simulink model "TwoTankSystem_continuous_controller"  (R2017a)
settings: Solver=ode4  StartTime=0.0  StopTime=SIM_TIME  FixedStep=STEP_SIZE  RelTol=1e-3  EnableMultiTasking=on
values from neighbouring files (symbols this model uses):
  At = 0.785    [TwoTankSystem.m]
  Av0 = 0.0122    [TwoTankSystem.m]
  Av1 = 1.2*0.0122    (= 0.01464)    [TwoTankSystem.m]
  B = B(:,1:2)    [TwoTankSystem.m]
  Bv = B(:,3:5)    [TwoTankSystem.m]
  C0 = 0.056    [TwoTankSystem.m]
  Dv = 2.66    [TwoTankSystem.m]
  K_CT = K_fs    [TwoTankSystem.m]
  ka = 0.004    [TwoTankSystem.m]
  kh = 2    [TwoTankSystem.m]
  kt = 0.1    [TwoTankSystem.m]
  r0 = [H_ref0 T_ref0]'    [TwoTankSystem.m]
  r1 = [0.5 -0.5]'    [TwoTankSystem.m]
  Tc = 1500    [TwoTankSystem.m]
  Tc0 = 30    [TwoTankSystem.m]
  Tc1 = 20    [TwoTankSystem.m]
  Tref1 = 100    [TwoTankSystem.m]
  Tref2 = 500    [TwoTankSystem.m]
  Tv = 2200    [TwoTankSystem.m]
  Tw = 300    [TwoTankSystem.m]
  Tw0 = 60    [TwoTankSystem.m]
  Tw1 = 75    [TwoTankSystem.m]
  u0 = u0(1:2,1)    [TwoTankSystem.m]
  v0 = u0(3:5,1)    [TwoTankSystem.m]
  x0 = xFinal'    [TwoTankSystem.m]
  x0_lin = zeros(size(A,1),1)    [TwoTankSystem.m]
  y0 = C*x0    [TwoTankSystem.m]
undefined symbols (not defined in the file or in its folder): A, C
settings Model: Creator=roga  LastModifiedBy=Roberto
settings DataIOCC: LimitDataPoints=on  SaveFinalState=on  SaveFormat=Array
settings OptimizationCC: LifeSpan=inf
settings DebuggingCC: UnderspecifiedInitializationDetection=Classic  MergeDetectMultiDrivingBlocksExec=none  SolverPrmCheckMsg=warning  StateNameClashWarn=warning  SFUnexpectedBacktrackingDiag=warning  SFNoUnconditionalDefaultTransitionDiag=warning  SFExecutionAtInitializationDiag=none
settings HardwareCC: ProdBitPerPointer=32  ProdBitPerSizeT=32  ProdBitPerPtrDiffT=32  ProdLargestAtomicFloat=None  ProdIntDivRoundTo=Undefined  ProdEndianess=Unspecified  ProdWordSize=32  ProdHWDeviceType=32-bit Generic
settings ModelReferenceCC: PropagateSignalLabelsOutOfModel=off
settings GRTTargetCC: TargetLangStandard=C89/C90 (ANSI)  GeneratePreprocessorConditionals=Disable all
settings ConfigComp: CovMetricSettings=dw  CovHtmlReporting=on  CovSaveCumulativeToWorkspaceVar=on  CovSaveSingleToWorkspaceVar=on  CovExternalEMLEnable=off  CovSFcnEnable=off

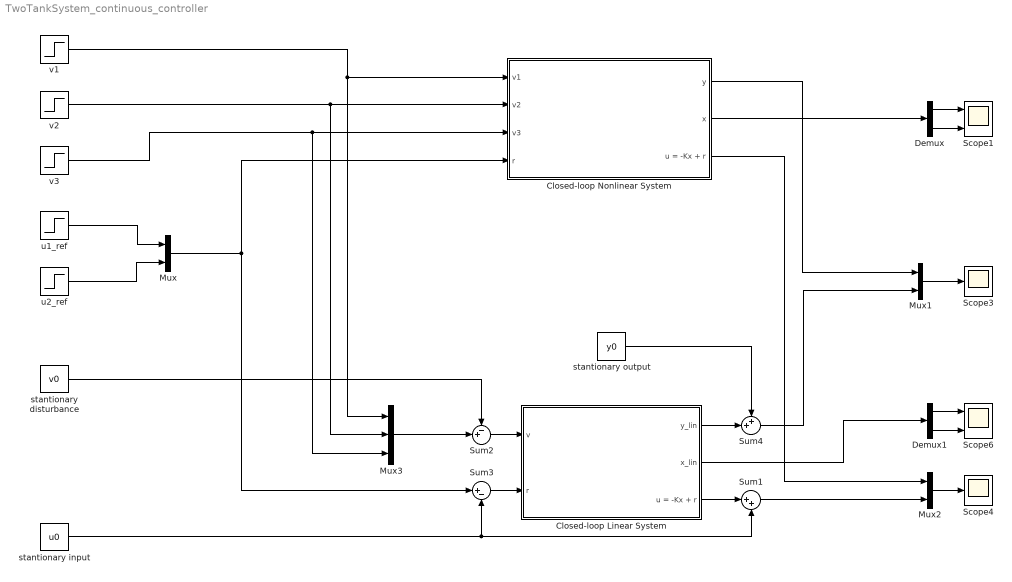
== system TwoTankSystem_continuous_controller ==
  Closed-loop Linear System : Subsystem
      mask Display:
      | port_label('output', 1, '\Delta y','texmode','on')
      | port_label('output', 2, '\Delta x','texmode','on')
      | port_label('output', 3, '\Delta u = - K \Delta x + \Delta r','texmode','on')
      | port_label('input', 1, '\Delta v','texmode','on')
      | port_label('input', 2, '\Delta r','texmode','on')
  Closed-loop Nonlinear System : Subsystem
  Demux : Demux  Outputs=2
  Demux1 : Demux  Outputs=2
  Mux : Mux  Inputs=2
  Mux1 : Mux  Inputs=2
  Mux2 : Mux  Inputs=2
  Mux3 : Mux  Inputs=3
  Scope1 : Scope  NumInputPorts=2
  Scope3 : Scope
  Scope4 : Scope
  Scope6 : Scope  NumInputPorts=2
  Sum1 : Sum  Inputs=|++
  Sum2 : Sum  Inputs=-+|
  Sum3 : Sum  Inputs=|+-
  Sum4 : Sum  Inputs=++|
  stantionary disturbance : Constant  Value=v0
  stantionary input : Constant  Value=u0
  stantionary output : Constant  Value=y0
  u1_ref : Step  Time=Tref1  Before=r0(1)+u0(1)  After=r1(1)+u0(1)  SampleTime=0
  u2_ref : Step  Time=Tref2  Before=r0(2)+u0(1)  After=r1(2)+u0(2)  SampleTime=0
  v1 : Step  Time=Tv+1000  Before=Av0  After=Av1  SampleTime=0
  v2 : Step  Time=Tw+1000  Before=Tw0  After=Tw1  SampleTime=0
  v3 : Step  Time=Tc+1000  Before=Tc0  After=Tc1  SampleTime=0
  wires:
  Demux/1 -> Scope1/1
  Demux/2 -> Scope1/2
  v1/1 -> Mux3/1, Closed-loop Nonlinear System/1(v1)
  v3/1 -> Mux3/3, Closed-loop Nonlinear System/3(v3)
  Mux1/1 -> Scope3/1
  v2/1 -> Mux3/2, Closed-loop Nonlinear System/2(v2)
  Sum2/1 -> Closed-loop Linear System/1(v)
  Mux3/1 -> Sum2/2
  stantionary disturbance/1 -> Sum2/1
  u1_ref/1 -> Mux/1
  u2_ref/1 -> Mux/2
  Mux/1 -> Closed-loop Nonlinear System/4(r), Sum3/1
  Sum3/1 -> Closed-loop Linear System/2(r)
  stantionary input/1 -> Sum1/2, Sum3/2
  Closed-loop Linear System/1(y_lin) -> Sum4/2
  stantionary output/1 -> Sum4/1
  Sum4/1 -> Mux1/2
  Closed-loop Nonlinear System/1(y) -> Mux1/1
  Closed-loop Nonlinear System/2(x) -> Demux/1
  Demux1/1 -> Scope6/1
  Demux1/2 -> Scope6/2
  Closed-loop Linear System/2(x_lin) -> Demux1/1
  Closed-loop Linear System/3(u = -Kx + r) -> Sum1/1
  Mux2/1 -> Scope4/1
  Closed-loop Nonlinear System/3(u = -Kx + r) -> Mux2/1
  Sum1/1 -> Mux2/2

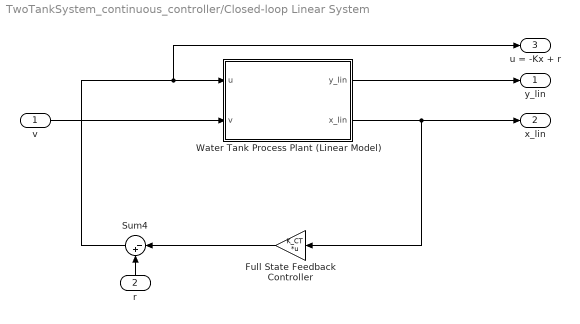
== system TwoTankSystem_continuous_controller/Closed-loop Linear System ==
  v : Inport
  r : Inport  Port=2
  Full State Feedback Controller : Gain  Gain=K_CT  Multiplication=Matrix(K*u) (u vector)
  Sum4 : Sum  Inputs=|-+
  Water Tank Process Plant (Linear Model) : Subsystem
      mask Display:
      | port_label('output',1,'y_{lin}','texmode','on')
      | port_label('output',2,'x_{lin}','texmode','on')
      | port_label('input',1,'u','texmode','on')
      | port_label('input',2,'v','texmode','on')
  y_lin : Outport
  x_lin : Outport  Port=2
  u = -Kx + r : Outport  Port=3
  wires:
  r/1 -> Sum4/2
  Full State Feedback Controller/1 -> Sum4/1
  Sum4/1 -> u = -Kx + r/1, Water Tank Process Plant (Linear Model)/1(u)
  Water Tank Process Plant (Linear Model)/2(x_lin) -> x_lin/1, Full State Feedback Controller/1
  Water Tank Process Plant (Linear Model)/1(y_lin) -> y_lin/1
  v/1 -> Water Tank Process Plant (Linear Model)/2(v)

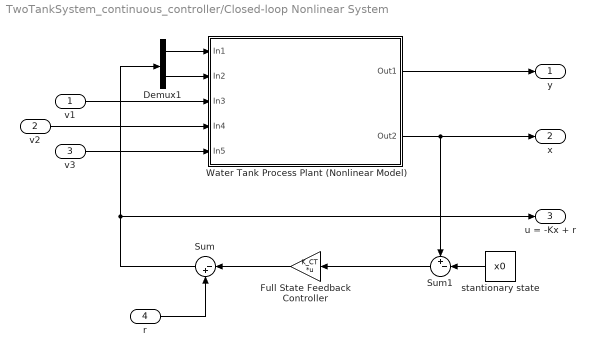
== system TwoTankSystem_continuous_controller/Closed-loop Nonlinear System ==
  v1 : Inport
  v2 : Inport  Port=2
  v3 : Inport  Port=3
  r : Inport  Port=4
  Demux1 : Demux  Outputs=2
  Full State Feedback Controller : Gain  Gain=K_CT  Multiplication=Matrix(K*u) (u vector)
  Sum : Sum  Inputs=|-+
  Sum1 : Sum  Inputs=+-|
  Water Tank Process Plant (Nonlinear Model) : Subsystem
      mask Display:
      | port_label('output',1,'y','texmode','on')
      | port_label('output',2,'x','texmode','on')
      | port_label('input',1,'u_1','texmode','on')
      | port_label('input',2,'u_2','texmode','on')
      | port_label('input',3,'A_v','texmode','on')
      | port_label('input',4,'T_w','texmode','on')
      | port_label('input',5,'T_c','texmode','on')
  stantionary state : Constant  Value=x0
  y : Outport
  x : Outport  Port=2
  u = -Kx + r : Outport  Port=3
  wires:
  v1/1 -> Water Tank Process Plant (Nonlinear Model)/3(In3)
  v2/1 -> Water Tank Process Plant (Nonlinear Model)/4(In4)
  v3/1 -> Water Tank Process Plant (Nonlinear Model)/5(In5)
  Full State Feedback Controller/1 -> Sum/1
  Demux1/1 -> Water Tank Process Plant (Nonlinear Model)/1(In1)
  Demux1/2 -> Water Tank Process Plant (Nonlinear Model)/2(In2)
  Sum1/1 -> Full State Feedback Controller/1
  stantionary state/1 -> Sum1/2
  Sum/1 -> Demux1/1, u = -Kx + r/1
  Water Tank Process Plant (Nonlinear Model)/2(Out2) -> x/1, Sum1/1
  Water Tank Process Plant (Nonlinear Model)/1(Out1) -> y/1
  r/1 -> Sum/2

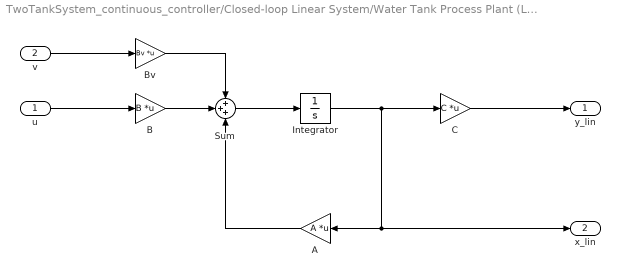
== system TwoTankSystem_continuous_controller/Closed-loop Linear System/Water Tank Process Plant (Linear Model) ==
  u : Inport
  v : Inport  Port=2
  A : Gain  Gain=A  Multiplication=Matrix(K*u) (u vector)
  B : Gain  Gain=B  Multiplication=Matrix(K*u) (u vector)
  Bv : Gain  Gain=Bv  Multiplication=Matrix(K*u) (u vector)
  C : Gain  Gain=C  Multiplication=Matrix(K*u) (u vector)
  Integrator : Integrator  InitialCondition=x0_lin
  Sum : Sum  Inputs=+++
  y_lin : Outport
  x_lin : Outport  Port=2
  wires:
  A/1 -> Sum/3
  B/1 -> Sum/2
  Bv/1 -> Sum/1
  Sum/1 -> Integrator/1
  Integrator/1 -> x_lin/1, A/1, C/1
  C/1 -> y_lin/1
  v/1 -> Bv/1
  u/1 -> B/1

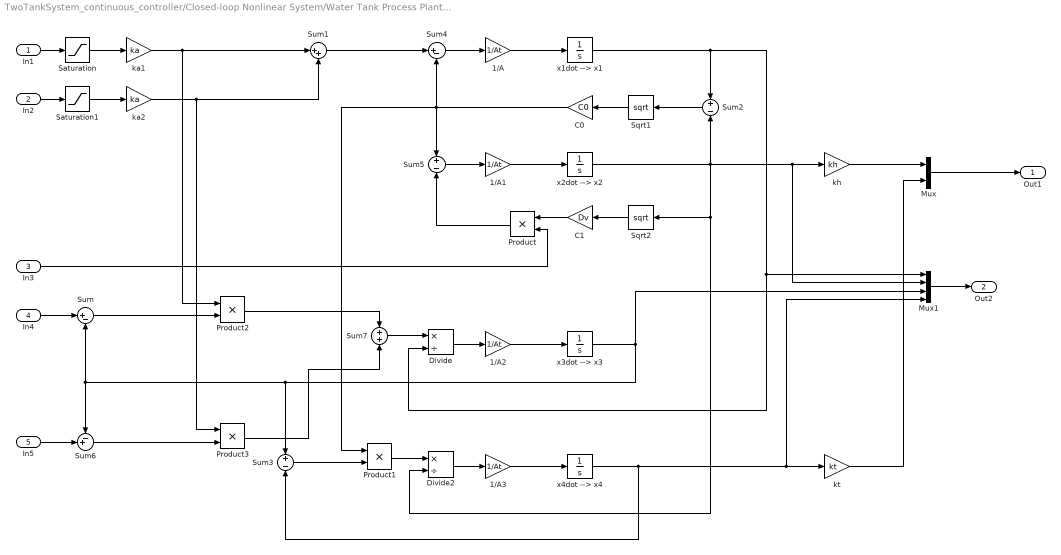
== system TwoTankSystem_continuous_controller/Closed-loop Nonlinear System/Water Tank Process Plant (Nonlinear Model) ==
  In1 : Inport
  In2 : Inport  Port=2
  In3 : Inport  Port=3
  In4 : Inport  Port=4
  In5 : Inport  Port=5
  1/A{,1..3} (4 alike) : Gain  Gain=1/At
  C0 : Gain  Gain=C0
  C1 : Gain  Gain=Dv
  Divide : Product  Inputs=*/
  Divide2 : Product  Inputs=*/
  Mux : Mux  Inputs=2
  Mux1 : Mux
  Product{,1..3} (4 alike) : Product
  Saturation : Saturate  UpperLimit=10  LowerLimit=0
  Saturation1 : Saturate  UpperLimit=10  LowerLimit=0
  Sqrt1 : Sqrt  SaturateOnIntegerOverflow=on
  Sqrt2 : Sqrt  SaturateOnIntegerOverflow=on
  Sum : Sum  Inputs=|+-
  Sum1 : Sum  Inputs=|++
  Sum2 : Sum  Inputs=+-
  Sum3 : Sum  Inputs=+-
  Sum4 : Sum  Inputs=|+-
  Sum5 : Sum  Inputs=+-
  Sum6 : Sum  Inputs=-+|
  Sum7 : Sum
  ka1 : Gain  Gain=ka
  ka2 : Gain  Gain=ka
  kh : Gain  Gain=kh
  kt : Gain  Gain=kt
  x1dot --> x1 : Integrator  InitialCondition=x0(1)  LimitOutput=on  LowerSaturationLimit=0
  x2dot --> x2 : Integrator  InitialCondition=x0(2)  LimitOutput=on  LowerSaturationLimit=0
  x3dot --> x3 : Integrator  InitialCondition=x0(3)
  x4dot --> x4 : Integrator  InitialCondition=x0(4)
  Out1 : Outport
  Out2 : Outport  Port=2
  wires:
  Product1/1 -> Divide2/1
  In2/1 -> Saturation1/1
  Divide/1 -> 1/A2/1
  Sum6/1 -> Product3/2
  In4/1 -> Sum/1
  1/A1/1 -> x2dot --> x2/1
  Sum5/1 -> 1/A1/1
  Product/1 -> Sum5/2
  x1dot --> x1/1 -> Sum2/1, Mux1/1, Divide/2
  Sum/1 -> Product2/2
  C1/1 -> Product/1
  Sum3/1 -> Product1/2
  Sqrt2/1 -> C1/1
  1/A2/1 -> x3dot --> x3/1
  In1/1 -> Saturation/1
  In3/1 -> Product/2
  kh/1 -> Mux/1
  x4dot --> x4/1 -> Mux1/4, kt/1, Sum3/2
  C0/1 -> Sum4/2, Product1/1, Sum5/1
  1/A3/1 -> x4dot --> x4/1
  x2dot --> x2/1 -> Mux1/2, kh/1, Divide2/2, Sqrt2/1, Sum2/2
  Divide2/1 -> 1/A3/1
  Sum7/1 -> Divide/1
  In5/1 -> Sum6/2
  Product2/1 -> Sum7/1
  Product3/1 -> Sum7/2
  Mux/1 -> Out1/1
  kt/1 -> Mux/2
  x3dot --> x3/1 -> Sum3/1, Sum6/1, Sum/2, Mux1/3
  1/A/1 -> x1dot --> x1/1
  Sum1/1 -> Sum4/1
  Mux1/1 -> Out2/1
  Sqrt1/1 -> C0/1
  Sum2/1 -> Sqrt1/1
  Sum4/1 -> 1/A/1
  ka1/1 -> Sum1/1, Product2/1
  ka2/1 -> Product3/1, Sum1/2
  Saturation/1 -> ka1/1
  Saturation1/1 -> ka2/1
